simulink model "PID_flam"  (R2017a)
settings: Solver=VariableStepAuto  StartTime=0.0  StopTime=10.0  RelTol=1e-3
libraries: simulink x1
settings Model: Creator=robotica  LastModifiedBy=robotica

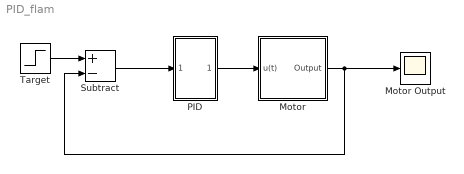
== system PID_flam ==
  Motor : Subsystem
  Motor Output : Scope
  PID : Subsystem
  Subtract : Sum  Inputs=+-
  Target : Step  SampleTime=1
  wires:
  PID/1(u(t)) -> Motor/1(u(t))
  Target/1 -> Subtract/1
  Subtract/1 -> PID/1(e(t))
  Motor/1(Output) -> Subtract/2, Motor Output/1

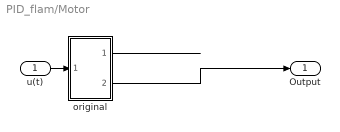
== system PID_flam/Motor ==
  u(t) : Inport
  original : Subsystem
  Output : Outport
  wires:
  u(t)/1 -> original/1(signal)
  original/1(noisy) -> ?
  original/2(clean) -> Output/1

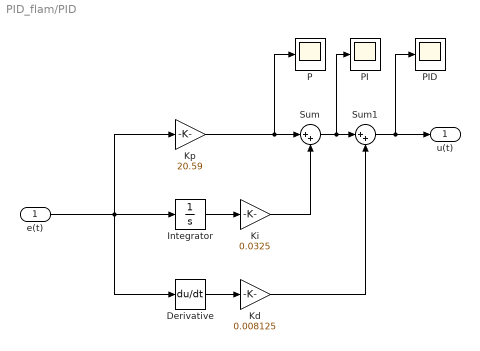
== system PID_flam/PID ==
  e(t) : Inport
  Derivative : Derivative
  Integrator : Integrator
  Kd : Gain  Gain=0.008125
  Ki : Gain  Gain=0.0325
  Kp : Gain  Gain=20.59
  P : Scope
  PI : Scope
  PID : Scope
  Sum : Sum  Inputs=|++
  Sum1 : Sum  Inputs=|++
  u(t) : Outport
  wires:
  Integrator/1 -> Ki/1
  Derivative/1 -> Kd/1
  Kp/1 -> P/1, Sum/1
  Ki/1 -> Sum/2
  Sum/1 -> PI/1, Sum1/1
  Kd/1 -> Sum1/2
  e(t)/1 -> Derivative/1, Kp/1, Integrator/1
  Sum1/1 -> u(t)/1, PID/1

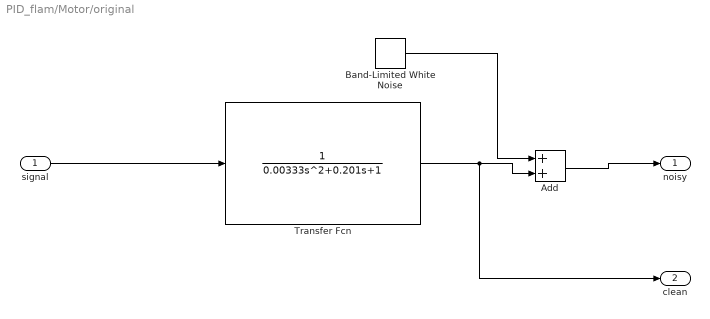
== system PID_flam/Motor/original ==
  signal : Inport
  Add : Sum
  Band-Limited White Noise : simulink/Sources/Band-Limited White Noise  Cov=[0.0000001]  Ts=0.001  seed=[23341]
  Transfer Fcn : TransferFcn  Denominator=[0.00333 0.201 1]
  noisy : Outport
  clean : Outport  Port=2
  wires:
  Transfer Fcn/1 -> clean/1, Add/2
  Band-Limited White Noise/1 -> Add/1
  Add/1 -> noisy/1
  signal/1 -> Transfer Fcn/1
